simulink model "assignment_mimo_2"  (R2020b)
settings: Solver=VariableStepAuto  StartTime=0.0  StopTime=600  RelTol=1e-3
undefined symbols (not defined in the file or in its folder): ctr_A, ctr_B, ctr_C, ctr_D, G_A, G_B, G_C, G_D, Gd_A, Gd_B, Gd_C, Gd_D
libraries: simulink x1
settings Model: Creator=long  LastModifiedBy=long
settings DataIOCC: ExternalInput=[t, d]

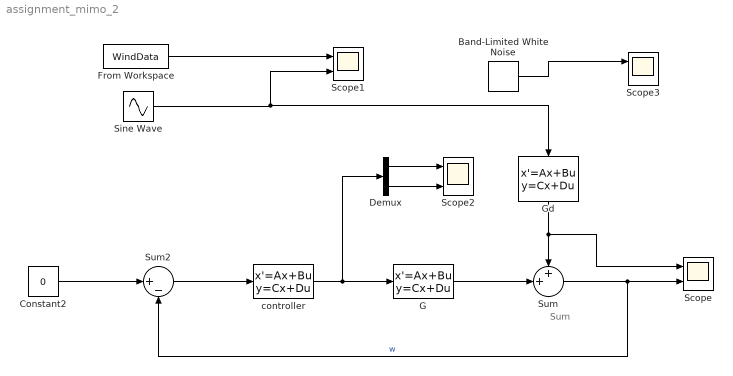
== system assignment_mimo_2 ==
  note: Sum
  Band-Limited White Noise : simulink/Sources/Band-Limited White Noise  Cov=[1]  Ts=0.01  seed=[23341]
  Constant2 : Constant  Value=0
  Demux : Demux  Outputs=2
  From Workspace : FromWorkspace  VariableName=WindData  SampleTime=0.01
  G : StateSpace  A=G_A  B=G_B  C=G_C  D=G_D  InitialCondition=0
  Gd : StateSpace  A=Gd_A  B=Gd_B  C=Gd_C  D=Gd_D  InitialCondition=0
  Scope{,1..3} (4 alike) : Scope  NumInputPorts=2
  Sine Wave : Sin  Amplitude=2  Frequency=0.002*pi  SampleTime=0
  Sum : Sum  Inputs=++|
  Sum2 : Sum  Inputs=|+-
  controller : StateSpace  A=ctr_A  B=ctr_B  C=ctr_C  D=ctr_D  InitialCondition=0
  wires:
  controller/1 -> Demux/1, G/1
  Constant2/1 -> Sum2/1
  Sum2/1 -> controller/1
  G/1 -> Sum/2
  Sum/1 -> Scope/2, Sum2/2  "w"
  From Workspace/1 -> Scope1/1
  Demux/1 -> Scope2/1
  Demux/2 -> Scope2/2
  Sine Wave/1 -> Gd/1, Scope1/2
  Band-Limited White Noise/1 -> Scope3/1
  Gd/1 -> Scope/1, Sum/1
